simulink model "temp_control_ecu"  (R2024a)
settings: Solver=VariableStepAuto  StartTime=0.0  StopTime=10.0  RelTol=1e-3
libraries: spsControlledVoltageSourceLib x1, spsDCMachineLib x1, spsDCVoltageSourceLib x1, simulink x1, spsVoltageMeasurementLib x1, sps_lib x1
settings Model: Creator=farza  LastModifiedBy=farza

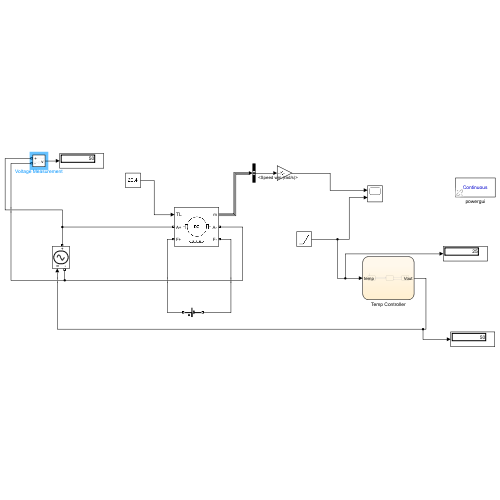
[thumbnail: Simulink's stored preview of the top-level diagram]
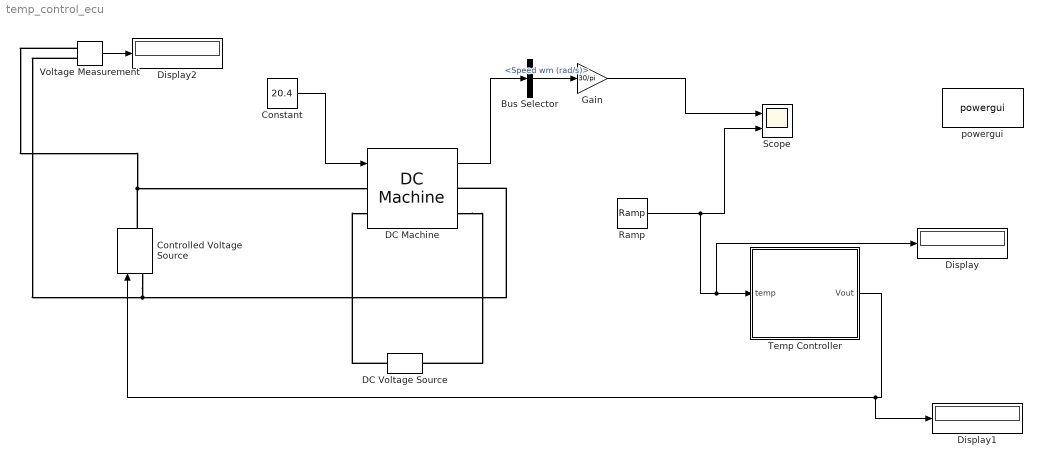
== system temp_control_ecu ==
  Bus Selector : BusSelector  OutputSignals=Speed wm (rad/s)
  Constant : Constant  Value=20.4
  Controlled Voltage Source : spsControlledVoltageSourceLib/Controlled Voltage Source  Initialize=on  Source_Type=DC  Amplitude=0  Phase=0  Frequency=0  Measurements=Voltage
  DC Machine : spsDCMachineLib/DC Machine  PresetModel=01: 5HP 240V 1750RPM Field:300V  MechanicalLoad=Torque TL  FieldType=Wound  ShowDetailedParameters=on  MeasurementBus=off  RLa=[2.581 0.028]  RLf=[281.2 156]  Laf=0.9483  MachineConstant=Torque constant (N.m/A)  Ke=1.8  Kt=1.8  J=0.02215  Bm=0.002953  Tf=0.5161  w0=1  Ifinit=1.06685633001422  TsPowergui=0  TsBlock=-1
  DC Voltage Source : spsDCVoltageSourceLib/DC Voltage Source  Amplitude=300  Measurements=None
  Display : Display
  Display1 : Display
  Display2 : Display
  Gain : Gain  Gain=30/pi
  Ramp : simulink/Sources/Ramp  slope=.5  start=0  InitialOutput=20
  Scope : Scope  NumInputPorts=2
  Temp Controller : Stateflow chart  TreatAsAtomicUnit=on
  Voltage Measurement : spsVoltageMeasurementLib/Voltage Measurement  PhasorSimulation=off  OutputType=Complex  PSBequivalent=0
  powergui : sps_lib/powergui  Priority=1  SimulationMode=Continuous  SampleTime=50e-6  frequency=60  Iterations=50  frequencyindice=0  Pbase=100e6  ErrMax=1e-4  UnitsV=kV  UnitsW=MW  buscounter=0  FunctionMessages=off  echomessages=off  EnableUseOfTLC=off  CurrentSourceSwitches=off  DisableSnubberDevices=off  DisableRonSwitches=off  DisableVfSwitches=off  DisplayEquations=off  AutomaticDiscreteSolvers=off  SolverType=Tustin/Backward Euler (TBE)  Interpol=off  ExternalGateDelay=off  methode=off  Ts=100  x0status=blocks  SPID=on  SwTol=0  HookPort=off  NonlinearTolerance=1e-4  nMaxIteration=100  ContinueOnMaxIteration=off  RestoreLinks=warning  ResistiveCurrentMeasurement=off  Frange=[0:2:500]  Ylog=off  Xlog=on  ShowGrid=off  save=off  variable=ZData  structure=0  ZoomFFT=off  StartTime=0.0  cycles=1  DisplayStyle=1  fundamental=60  FreqAxis=off  MaxFrequency=1000  frequencyindicesteady=1  RmsSteady=1  display=off
  wires:
  Constant/1 -> DC Machine/1
  DC Machine/1 -> Bus Selector/1
  Bus Selector/1 -> Gain/1  "<Speed wm (rad/s)>"
  Gain/1 -> Scope/1
  Temp Controller/1(Vout) -> Display1/1, Controlled Voltage Source/1
  Ramp/1 -> Display/1, Temp Controller/1(temp), Scope/2
  Voltage Measurement/1 -> Display2/1
  connections:
  DC Voltage Source/RConn1 -- DC Machine/LConn2
  DC Machine/RConn2 -- DC Voltage Source/LConn1
  Controlled Voltage Source/RConn1 -- DC Machine/LConn1 -- Voltage Measurement/LConn1
  Controlled Voltage Source/LConn1 -- DC Machine/RConn1 -- Voltage Measurement/LConn2

== stateflow chart temp_control_ecu/Temp Controller ==
  state COOL_LOW
    Vout=50
  state COOL_MED
    entry:
    Vout=100
  state COOL_HIGH
    entry:
    Vout=240
  (default) -> COOL_LOW
  COOL_MED -> COOL_HIGH [order 2] : [temp>=60]
  COOL_LOW -> COOL_MED : [temp>=30]
  COOL_MED -> COOL_LOW [order 1] : [temp<30]
  COOL_HIGH -> COOL_MED : [temp<60]
  data: temp input; Vout output
